simulink model "testNoiseIMU"  (R2021a)
settings: Solver=VariableStepAuto  StartTime=0.0  StopTime=3600  RelTol=1e-3
undefined symbols (not defined in the file or in its folder): noiseAcc, noiseAng
libraries: simulink x2
settings Model: Creator=jmher  LastModifiedBy=jmher

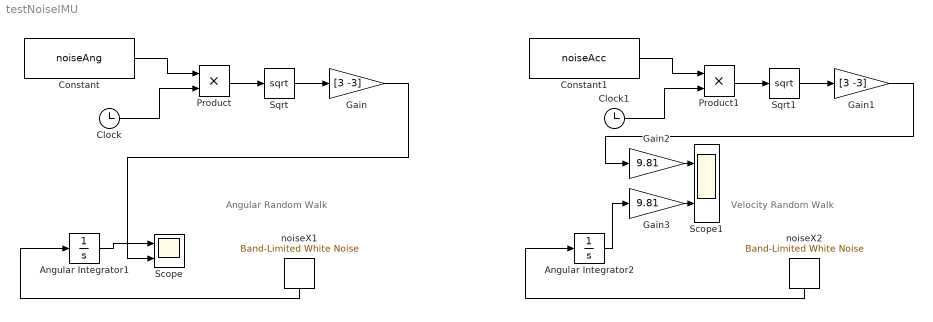
== system testNoiseIMU ==
  note: Angular Random Walk
  note: Velocity Random Walk
  Angular Integrator1 : Integrator
  Angular Integrator2 : Integrator
  Clock : Clock
  Clock1 : Clock
  Constant : Constant  Value=noiseAng
  Constant1 : Constant  Value=noiseAcc
  Gain : Gain  Gain=[3 -3]
  Gain1 : Gain  Gain=[3 -3]
  Gain2 : Gain  Gain=9.81
  Gain3 : Gain  Gain=9.81
  Product : Product
  Product1 : Product
  Scope : Scope  NumInputPorts=2
  Scope1 : Scope  NumInputPorts=2
  Sqrt : Sqrt  SaturateOnIntegerOverflow=on
  Sqrt1 : Sqrt  SaturateOnIntegerOverflow=on
  noiseX1 : simulink/Sources/Band-Limited White Noise  Cov=noiseAng  Ts=1/40  seed=randi(1000,100,1)
  noiseX2 : simulink/Sources/Band-Limited White Noise  Cov=noiseAcc  Ts=1/40  seed=randi(1000,100,1)
  wires:
  noiseX1/1 -> Angular Integrator1/1
  Constant/1 -> Product/1
  Clock/1 -> Product/2
  Product/1 -> Sqrt/1
  Sqrt/1 -> Gain/1
  Gain/1 -> Scope/2
  Angular Integrator1/1 -> Scope/1
  Product1/1 -> Sqrt1/1
  noiseX2/1 -> Angular Integrator2/1
  Sqrt1/1 -> Gain1/1
  Constant1/1 -> Product1/1
  Clock1/1 -> Product1/2
  Gain2/1 -> Scope1/1
  Gain3/1 -> Scope1/2
  Angular Integrator2/1 -> Gain3/1
  Gain1/1 -> Gain2/1
